simulink model "Engine_Propeller_Table_Model_SAAM"  (R2018a)
settings: Solver=FixedStepAuto  StartTime=0.0  StopTime=10.0  FixedStep=dt  RelTol=1e-3
values from neighbouring files (symbols this model uses):
  airDensityBreakPoints_eng = linspace(0.0006, 0.0027, 4)    [airplane_ic_constants.m]
  casBreakpoints_eng = 0:50:300    [airplane_ic_constants.m]
  engine_tables =     [engine_tables.mat]
  powerBreakpoints_eng = linspace(0, P_e_max, 4)    [airplane_ic_constants.m]
settings Model: Creator=Kyle  LastModifiedBy=Kyle

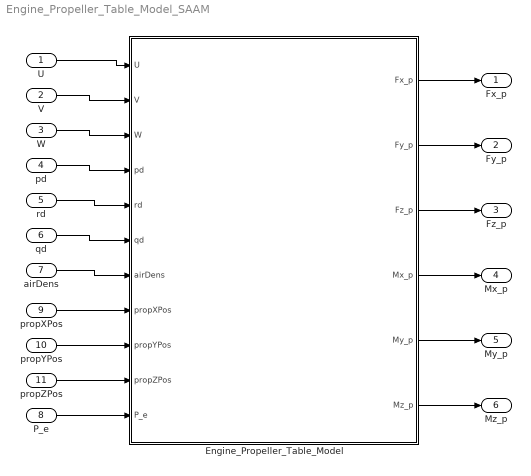
== system Engine_Propeller_Table_Model_SAAM ==
  U : Inport
  V : Inport  Port=2
  W : Inport  Port=3
  pd : Inport  Port=4
  rd : Inport  Port=5
  qd : Inport  Port=6
  airDens : Inport  Port=7
  P_e : Inport  Port=8
  propXPos : Inport  Port=9
  propYPos : Inport  Port=10
  propZPos : Inport  Port=11
  Engine_Propeller_Table_Model : Subsystem
  Fx_p : Outport
  Fy_p : Outport  Port=2
  Fz_p : Outport  Port=3
  Mx_p : Outport  Port=4
  My_p : Outport  Port=5
  Mz_p : Outport  Port=6
  wires:
  U/1 -> Engine_Propeller_Table_Model/1(U)
  V/1 -> Engine_Propeller_Table_Model/2(V)
  W/1 -> Engine_Propeller_Table_Model/3(W)
  pd/1 -> Engine_Propeller_Table_Model/4(pd)
  propXPos/1 -> Engine_Propeller_Table_Model/8(propXPos)
  propYPos/1 -> Engine_Propeller_Table_Model/9(propYPos)
  propZPos/1 -> Engine_Propeller_Table_Model/10(propZPos)
  P_e/1 -> Engine_Propeller_Table_Model/11(P_e)
  rd/1 -> Engine_Propeller_Table_Model/5(rd)
  qd/1 -> Engine_Propeller_Table_Model/6(qd)
  airDens/1 -> Engine_Propeller_Table_Model/7(airDens)
  Engine_Propeller_Table_Model/4(Mx_p) -> Mx_p/1
  Engine_Propeller_Table_Model/6(Mz_p) -> Mz_p/1
  Engine_Propeller_Table_Model/5(My_p) -> My_p/1
  Engine_Propeller_Table_Model/2(Fy_p) -> Fy_p/1
  Engine_Propeller_Table_Model/1(Fx_p) -> Fx_p/1
  Engine_Propeller_Table_Model/3(Fz_p) -> Fz_p/1

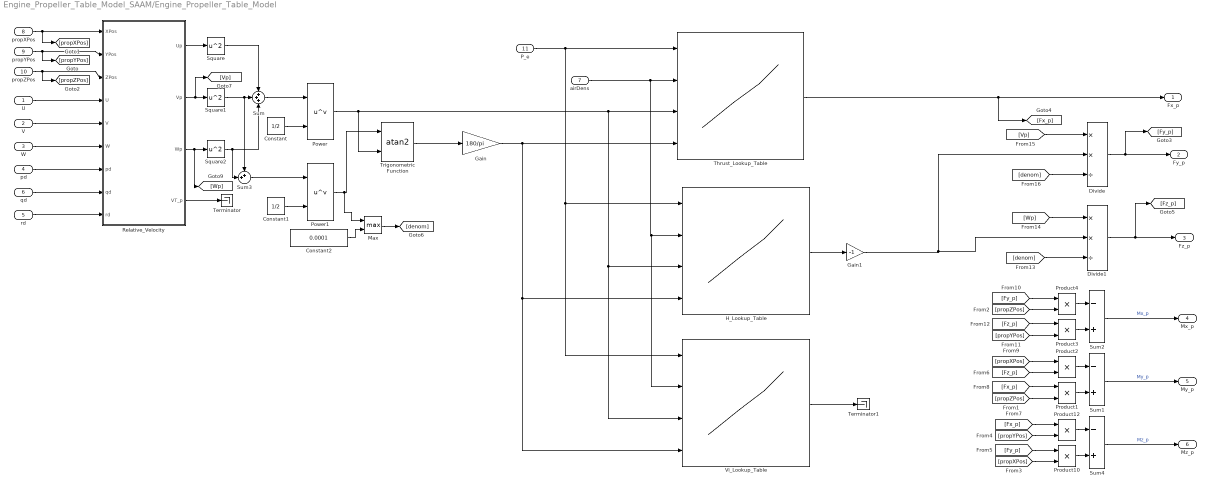
== system Engine_Propeller_Table_Model_SAAM/Engine_Propeller_Table_Model ==
  U : Inport
  V : Inport  Port=2
  W : Inport  Port=3
  pd : Inport  Port=4
  rd : Inport  Port=5
  qd : Inport  Port=6
  airDens : Inport  Port=7
  propXPos : Inport  Port=8
  propYPos : Inport  Port=9
  propZPos : Inport  Port=10
  P_e : Inport  Port=11
  Constant : Constant  Value=1/2
  Constant1 : Constant  Value=1/2
  Constant2 : Constant  Value=0.0001
  Divide : Product  Inputs=**/
  Divide1 : Product  Inputs=**/
  Gain : Gain  Gain=180/pi
  Gain1 : Gain  Gain=-1
  H_Lookup_Table : Lookup_n-D  NumberOfTableDimensions=4  LookupTableObject=''  BreakpointsForDimension1=powerBreakpoints_eng  BreakpointsForDimension2=airDensityBreakPoints_eng  BreakpointsForDimension3=casBreakpoints_eng  BreakpointsForDimension4=angleBreakPoints_eng  BreakpointsForDimension1FirstPoint=10  BreakpointsForDimension2FirstPoint=10  BreakpointsForDimension1Spacing=12  BreakpointsForDimension2Spacing=12  IndexSearchMethod=Linear search  BeginIndexSearchUsingPreviousIndexResult=on  Table=engine_tables.H(:,:,:,:)  DiagnosticForOutOfRangeInput=Error  InternalRulePriority=Speed  RndMeth=Simplest  InputSameDT=on
  Max : MinMax  Function=max  Inputs=2
  Power : Math  Operator=pow  SaturateOnIntegerOverflow=on
  Power1 : Math  Operator=pow  SaturateOnIntegerOverflow=on
  Product{1..4,10,12} (6 alike) : Product
  Relative_Velocity : Subsystem
  Square : Math  Operator=square  SaturateOnIntegerOverflow=on
  Square1 : Math  Operator=square  SaturateOnIntegerOverflow=on
  Square2 : Math  Operator=square  SaturateOnIntegerOverflow=on
  Sum : Sum  Inputs=+++
  Sum1 : Sum  Inputs=-+
  Sum2 : Sum  Inputs=-+
  Sum3 : Sum  Inputs=++|
  Sum4 : Sum  Inputs=-+
  Terminator : Terminator
  Terminator1 : Terminator
  Thrust_Lookup_Table : Lookup_n-D  NumberOfTableDimensions=4  LookupTableObject=''  BreakpointsForDimension1=powerBreakpoints_eng  BreakpointsForDimension2=airDensityBreakPoints_eng  BreakpointsForDimension3=casBreakpoints_eng  BreakpointsForDimension4=angleBreakPoints_eng  BreakpointsForDimension1FirstPoint=10  BreakpointsForDimension2FirstPoint=10  BreakpointsForDimension1Spacing=12  BreakpointsForDimension2Spacing=12  IndexSearchMethod=Linear search  BeginIndexSearchUsingPreviousIndexResult=on  Table=engine_tables.T(:,:,:,:)  DiagnosticForOutOfRangeInput=Error  InternalRulePriority=Speed  RndMeth=Simplest  InputSameDT=on
  Trigonometric Function : Trigonometry  Operator=atan2
  Vi_Lookup_Table : Lookup_n-D  NumberOfTableDimensions=4  LookupTableObject=''  BreakpointsForDimension1=powerBreakpoints_eng  BreakpointsForDimension2=airDensityBreakPoints_eng  BreakpointsForDimension3=casBreakpoints_eng  BreakpointsForDimension4=angleBreakPoints_eng  BreakpointsForDimension1FirstPoint=10  BreakpointsForDimension2FirstPoint=10  BreakpointsForDimension1Spacing=12  BreakpointsForDimension2Spacing=12  IndexSearchMethod=Linear search  BeginIndexSearchUsingPreviousIndexResult=on  Table=engine_tables.vi(:,:,:,:)  DiagnosticForOutOfRangeInput=Error  InternalRulePriority=Speed  RndMeth=Simplest  InputSameDT=on
  Fx_p : Outport
  Fy_p : Outport  Port=2
  Fz_p : Outport  Port=3
  Mx_p : Outport  Port=4
  My_p : Outport  Port=5
  Mz_p : Outport  Port=6
  wires:
  propYPos/1 -> [propYPos], Relative_Velocity/2(YPos)
  propZPos/1 -> [propZPos], Relative_Velocity/3(ZPos)
  U/1 -> Relative_Velocity/4(U)
  V/1 -> Relative_Velocity/5(V)
  W/1 -> Relative_Velocity/6(W)
  pd/1 -> Relative_Velocity/7(pd)
  rd/1 -> Relative_Velocity/9(rd)
  qd/1 -> Relative_Velocity/8(qd)
  propXPos/1 -> [propXPos], Relative_Velocity/1(XPos)
  [propZPos] -> Product1/2
  Product12/1 -> Sum4/1
  Sum4/1 -> Mz_p/1  "Mz_p"
  [propYPos] -> Product12/2
  Product10/1 -> Sum4/2
  [propXPos] -> Product10/2
  Relative_Velocity/4(VT_p) -> Terminator/1
  [propZPos] -> Product4/2
  [Fy_p] -> Product10/1
  [Fx_p] -> Product12/1
  Product1/1 -> Sum1/2
  Product2/1 -> Sum1/1
  Sum1/1 -> My_p/1  "My_p"
  [Fx_p] -> Product1/1
  [Fz_p] -> Product2/2
  [propXPos] -> Product2/1
  Product4/1 -> Sum2/1
  Sum2/1 -> Mx_p/1  "Mx_p"
  Product3/1 -> Sum2/2
  [Fy_p] -> Product4/1
  [propYPos] -> Product3/2
  [Fz_p] -> Product3/1
  Vi_Lookup_Table/1 -> Terminator1/1
  airDens/1 -> Vi_Lookup_Table/2, H_Lookup_Table/2, Thrust_Lookup_Table/2
  P_e/1 -> Vi_Lookup_Table/1, H_Lookup_Table/1, Thrust_Lookup_Table/1
  Relative_Velocity/1(Up) -> Square/1
  Relative_Velocity/3(Wp) -> [Wp], Square2/1
  Square/1 -> Sum/1
  Square1/1 -> Sum3/1, Sum/2
  Square2/1 -> Sum3/2, Sum/3
  Constant/1 -> Power/2
  Sum/1 -> Power/1
  Power/1 -> Trigonometric Function/2, Vi_Lookup_Table/3, H_Lookup_Table/3, Thrust_Lookup_Table/3
  Sum3/1 -> Power1/1
  Constant1/1 -> Power1/2
  Power1/1 -> Max/1, Trigonometric Function/1
  Trigonometric Function/1 -> Gain/1
  Gain/1 -> Vi_Lookup_Table/4, H_Lookup_Table/4, Thrust_Lookup_Table/4
  Thrust_Lookup_Table/1 -> [Fx_p], Fx_p/1
  Relative_Velocity/2(Vp) -> [Vp], Square1/1
  H_Lookup_Table/1 -> Gain1/1
  Divide1/1 -> [Fz_p], Fz_p/1
  Divide/1 -> [Fy_p], Fy_p/1
  [Wp] -> Divide1/1
  [Vp] -> Divide/1
  Gain1/1 -> Divide1/2, Divide/2
  [denom] -> Divide/3
  [denom] -> Divide1/3
  Constant2/1 -> Max/2
  Max/1 -> [denom]

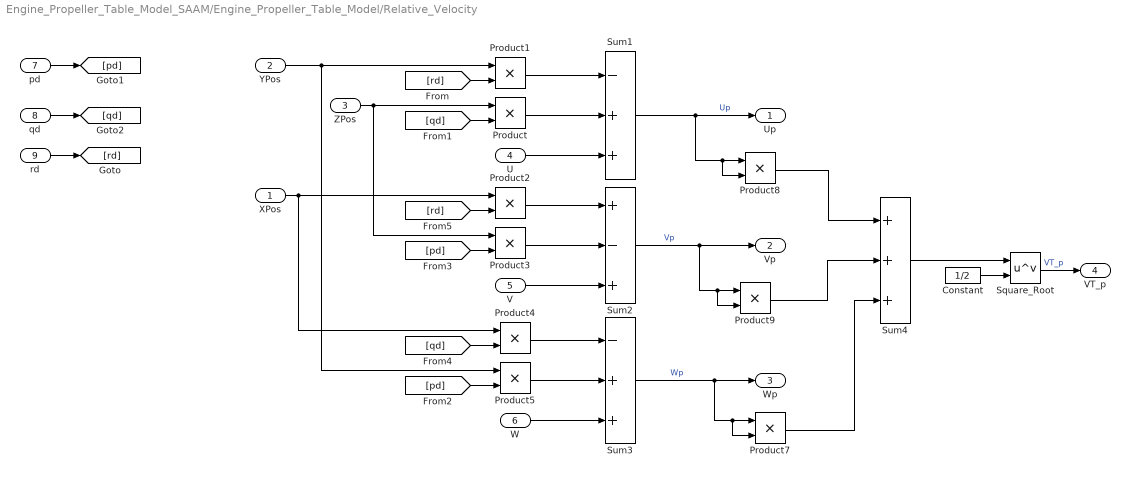
== system Engine_Propeller_Table_Model_SAAM/Engine_Propeller_Table_Model/Relative_Velocity ==
  XPos : Inport
  YPos : Inport  Port=2
  ZPos : Inport  Port=3
  U : Inport  Port=4
  V : Inport  Port=5
  W : Inport  Port=6
  pd : Inport  Port=7
  qd : Inport  Port=8
  rd : Inport  Port=9
  Constant : Constant  Value=1/2
  Product{,1..5,7..9} (9 alike) : Product
  Square_Root : Math  Operator=pow  SaturateOnIntegerOverflow=on
  Sum1 : Sum  Inputs=-++
  Sum2 : Sum  Inputs=+-+
  Sum3 : Sum  Inputs=-++
  Sum4 : Sum  Inputs=+++
  Up : Outport
  Vp : Outport  Port=2
  Wp : Outport  Port=3
  VT_p : Outport  Port=4
  wires:
  ZPos/1 -> Product3/1, Product/1
  Product/1 -> Sum1/2
  U/1 -> Sum1/3
  [rd] -> Product1/2
  Product1/1 -> Sum1/1
  rd/1 -> [rd]
  pd/1 -> [pd]
  qd/1 -> [qd]
  [qd] -> Product/2
  V/1 -> Sum2/3
  Sum3/1 -> Product7/2, Product7/1, Wp/1  "Wp"
  W/1 -> Sum3/3
  Product3/1 -> Sum2/2
  Product2/1 -> Sum2/1
  XPos/1 -> Product4/1, Product2/1
  YPos/1 -> Product5/1, Product1/1
  Product5/1 -> Sum3/2
  Product4/1 -> Sum3/1
  [pd] -> Product5/2
  [pd] -> Product3/2
  [rd] -> Product2/2
  [qd] -> Product4/2
  Sum1/1 -> Product8/2, Product8/1, Up/1  "Up"
  Sum2/1 -> Product9/1, Product9/2, Vp/1  "Vp"
  Square_Root/1 -> VT_p/1  "VT_p"
  Constant/1 -> Square_Root/2
  Sum4/1 -> Square_Root/1
  Product8/1 -> Sum4/1
  Product9/1 -> Sum4/2
  Product7/1 -> Sum4/3
